simulink library "cdsRio"  (Simulink 7.2)
settings: Solver=ode45  SolverMode=SingleTasking  StartTime=0.0  StopTime=10.0  RelTol=1e-3
libraries: simulink x1
settings Model: Creator=aivanov  LastModifiedBy=aivanov  ExtModeAutoUpdateStatusClock=off

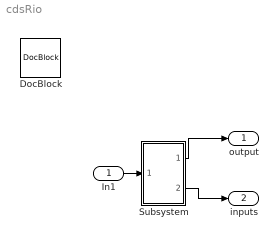
== system cdsRio ==
  In1 : Inport  OutDataType=sfix(16)  OutScaling=2^0
  DocBlock : simulink/Model-Wide Utilities/DocBlock  Tag="About \"inputs\" and \"outputs\""  SystemSampleTime=-1  DocumentType=Text
      content=|
      | It is possible to read the state of current digital outputs of the board
      | by using "outputs" or the second output line.
      |
      | "inputs" (port 2) has the digital inputs.
      settings: AttributesFormatString=%<Tag>
  Subsystem : Subsystem
  output : Outport  OutDataType=sfix(16)  OutScaling=2^0
  inputs : Outport  Port=2  OutDataType=sfix(16)  OutScaling=2^0
  wires:
  Subsystem/1(Out1) -> output/1
  In1/1 -> Subsystem/1(In1)
  Subsystem/2(Out2) -> inputs/1

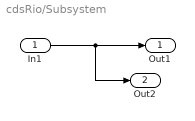
== system cdsRio/Subsystem ==
  In1 : Inport  OutDataType=sfix(16)  OutScaling=2^0
  Out1 : Outport  OutDataType=sfix(16)  OutScaling=2^0
  Out2 : Outport  Port=2  OutDataType=sfix(16)  OutScaling=2^0
  wires:
  In1/1 -> Out1/1, Out2/1
